simulink model "SIRobs"  (R2020a)
settings: Solver=VariableStepAuto  StartTime=0.0  StopTime=100  MaxStep=1e-2  RelTol=1e-3
values from neighbouring files (symbols this model uses):
  beta = X(1)    [ErroQuadratico.m]    (also in ErroQuadraticoSIR.m)
  I0 = 2    [ErroQuadratico.m]    (also in ErroQuadraticoSIR.m)
  r = X(2)    [ErroQuadratico.m]    (also in ErroQuadraticoSIR.m)
  R0 = 0    [ErroQuadratico.m]    (also in ErroQuadraticoSIR.m)
  S0 = 60e6    (= 60000000)    [ErroQuadratico.m]    (also in ErroQuadraticoSIR.m)
undefined symbols (not defined in the file or in its folder): beta0, I0o, l1, l2, p1, p2, r0, R0o, S0o
settings Model: Creator=a1  LastModifiedBy=a1

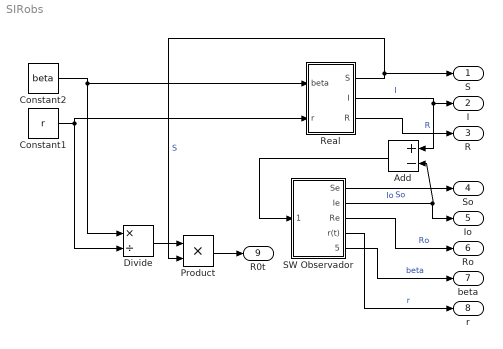
== system SIRobs ==
  Add : Sum  Inputs=+-
  Constant1 : Constant  Value=r
  Constant2 : Constant  Value=beta
  Divide : Product  Inputs=*/
  Product : Product
  Real : Subsystem
  SW Observador : Subsystem
  S : Outport
  I : Outport  Port=2
  R : Outport  Port=3
  So : Outport  Port=4
  Io : Outport  Port=5
  Ro : Outport  Port=6
  beta : Outport  Port=7
  r : Outport  Port=8
  R0t : Outport  Port=9
  wires:
  Constant1/1 -> Divide/2, Real/2(r)
  Add/1 -> SW Observador/1((y-ye))
  SW Observador/2(Ie) -> Io/1, Add/2  "Io"
  Real/2(I) -> Add/1, I/1  "I"
  Real/1(S) -> Product/2, S/1  "S"
  Real/3(R) -> R/1  "R"
  SW Observador/1(Se) -> So/1  "So"
  SW Observador/3(Re) -> Ro/1  "Ro"
  SW Observador/5(beta(t)) -> beta/1  "beta"
  SW Observador/4(r(t)) -> r/1  "r"
  Constant2/1 -> Divide/1, Real/1(beta)
  Divide/1 -> Product/1
  Product/1 -> R0t/1

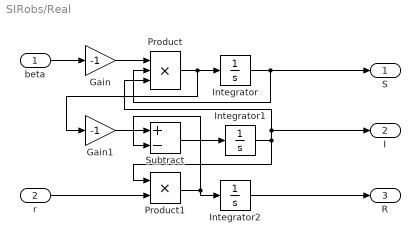
== system SIRobs/Real ==
  beta : Inport
  r : Inport  Port=2
  Gain : Gain  Gain=-1
  Gain1 : Gain  Gain=-1
  Integrator : Integrator  InitialCondition=S0
  Integrator1 : Integrator  InitialCondition=I0
  Integrator2 : Integrator  InitialCondition=R0
  Product : Product  Inputs=3
  Product1 : Product
  Subtract : Sum  Inputs=+-
  S : Outport
  I : Outport  Port=2
  R : Outport  Port=3
  wires:
  beta/1 -> Gain/1
  Gain1/1 -> Subtract/1
  Integrator2/1 -> R/1
  Gain/1 -> Product/1
  Product1/1 -> Integrator2/1, Subtract/2
  Subtract/1 -> Integrator1/1
  Product/1 -> Gain1/1, Integrator/1
  r/1 -> Product1/2
  Integrator/1 -> S/1, Product/2
  Integrator1/1 -> Product1/1, I/1, Product/3

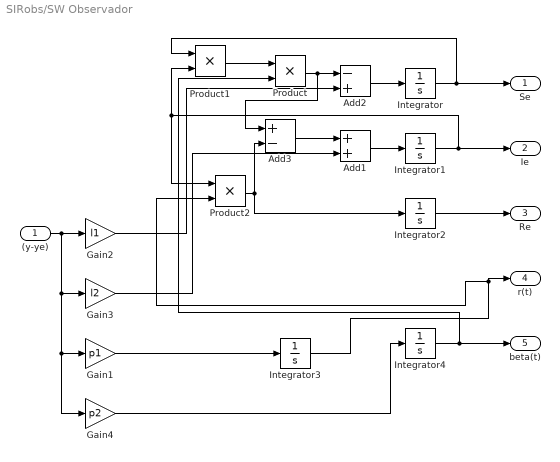
== system SIRobs/SW Observador ==
  (y-ye) : Inport
  Add1 : Sum
  Add2 : Sum  Inputs=-+
  Add3 : Sum  Inputs=+-
  Gain1 : Gain  Gain=p1
  Gain2 : Gain  Gain=l1
  Gain3 : Gain  Gain=l2
  Gain4 : Gain  Gain=p2
  Integrator : Integrator  InitialCondition=S0o
  Integrator1 : Integrator  InitialCondition=I0o
  Integrator2 : Integrator  InitialCondition=R0o
  Integrator3 : Integrator  InitialCondition=r0
  Integrator4 : Integrator  InitialCondition=beta0
  Product : Product
  Product1 : Product
  Product2 : Product
  Se : Outport
  Ie : Outport  Port=2
  Re : Outport  Port=3
  r(t) : Outport  Port=4
  beta(t) : Outport  Port=5
  wires:
  Integrator2/1 -> Re/1
  Integrator/1 -> Product1/1, Se/1
  Integrator1/1 -> Product2/1, Product1/2, Ie/1
  (y-ye)/1 -> Gain4/1, Gain1/1, Gain3/1, Gain2/1
  Product2/1 -> Integrator2/1, Add3/2
  Product/1 -> Add3/1, Add2/1
  Add2/1 -> Integrator/1
  Gain2/1 -> Add2/2
  Product1/1 -> Product/1
  Integrator4/1 -> Product/2, beta(t)/1
  Add1/1 -> Integrator1/1
  Gain3/1 -> Add1/2
  Add3/1 -> Add1/1
  Gain4/1 -> Integrator4/1
  Integrator3/1 -> Product2/2, r(t)/1
  Gain1/1 -> Integrator3/1
